simulink library "ESPA_lib"  (Simulink 7.5)
settings: Solver=ode45  StartTime=0.0  StopTime=10.0  RelTol=1e-3
values from neighbouring files (symbols this model uses):
  pESPA_bool_ToESPTrqSel_C = Simulink.Parameter    [ESPA_par.m]
  pESPA_cnt_TQDTrqDelyTi_C = Simulink.Parameter    [ESPA_par.m]
  pESPA_Nm_TMMinusTrq_C = Simulink.Parameter    [ESPA_par.m]
  pESPA_Nm_TMZeorTrq_C = Simulink.Parameter    [ESPA_par.m]
  pESPA_ratio_VehI_C = Simulink.Parameter    [ESPA_par.m]
  pESPA_rpm_TMZeroSpd_C = Simulink.Parameter    [ESPA_par.m]
libraries: BaseOperationLib_Browser x84
settings Model: Creator=wuaibin  LastModifiedBy=wuaibin

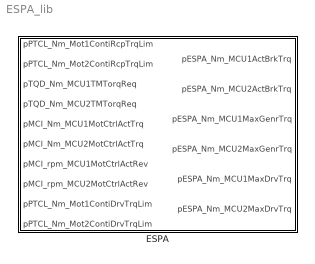
== system ESPA_lib ==
  ESPA : Subsystem

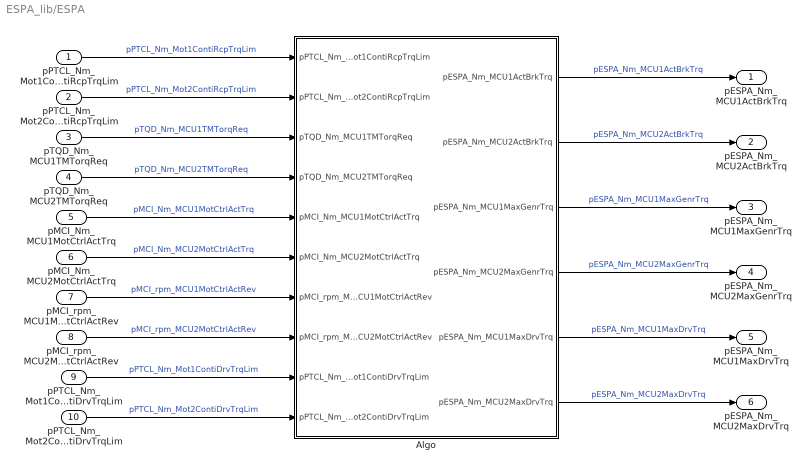
== system ESPA_lib/ESPA ==
  pPTCL_Nm_Mot1ContiRcpTrqLim : Inport
  pPTCL_Nm_Mot2ContiRcpTrqLim : Inport  Port=2
  pTQD_Nm_MCU1TMTorqReq : Inport  Port=3
  pTQD_Nm_MCU2TMTorqReq : Inport  Port=4
  pMCI_Nm_MCU1MotCtrlActTrq : Inport  Port=5
  pMCI_Nm_MCU2MotCtrlActTrq : Inport  Port=6
  pMCI_rpm_MCU1MotCtrlActRev : Inport  Port=7  OutDataType=fixdt(1, 16)  OutScaling=2^0
  pMCI_rpm_MCU2MotCtrlActRev : Inport  Port=8  OutDataType=fixdt(1, 16)  OutScaling=2^0
  pPTCL_Nm_Mot1ContiDrvTrqLim : Inport  Port=9
  pPTCL_Nm_Mot2ContiDrvTrqLim : Inport  Port=10
  Algo : Subsystem
  pESPA_Nm_MCU1ActBrkTrq : Outport  OutDataType=fixdt(1, 16)  OutScaling=2^0
  pESPA_Nm_MCU2ActBrkTrq : Outport  Port=2  OutDataType=fixdt(1, 16)  OutScaling=2^0
  pESPA_Nm_MCU1MaxGenrTrq : Outport  Port=3  OutDataType=fixdt(1, 16)  OutScaling=2^0
  pESPA_Nm_MCU2MaxGenrTrq : Outport  Port=4  OutDataType=fixdt(1, 16)  OutScaling=2^0
  pESPA_Nm_MCU1MaxDrvTrq : Outport  Port=5  OutDataType=fixdt(1, 16)  OutScaling=2^0
  pESPA_Nm_MCU2MaxDrvTrq : Outport  Port=6  OutDataType=fixdt(1, 16)  OutScaling=2^0
  wires:
  Algo/6(pESPA_Nm_MCU2MaxDrvTrq) -> pESPA_Nm_MCU2MaxDrvTrq/1  "pESPA_Nm_MCU2MaxDrvTrq"
  Algo/5(pESPA_Nm_MCU1MaxDrvTrq) -> pESPA_Nm_MCU1MaxDrvTrq/1  "pESPA_Nm_MCU1MaxDrvTrq"
  pPTCL_Nm_Mot2ContiDrvTrqLim/1 -> Algo/10(pPTCL_Nm_Mot2ContiDrvTrqLim)  "pPTCL_Nm_Mot2ContiDrvTrqLim"
  pPTCL_Nm_Mot1ContiDrvTrqLim/1 -> Algo/9(pPTCL_Nm_Mot1ContiDrvTrqLim)  "pPTCL_Nm_Mot1ContiDrvTrqLim"
  Algo/4(pESPA_Nm_MCU2MaxGenrTrq) -> pESPA_Nm_MCU2MaxGenrTrq/1  "pESPA_Nm_MCU2MaxGenrTrq"
  Algo/3(pESPA_Nm_MCU1MaxGenrTrq) -> pESPA_Nm_MCU1MaxGenrTrq/1  "pESPA_Nm_MCU1MaxGenrTrq"
  Algo/2(pESPA_Nm_MCU2ActBrkTrq) -> pESPA_Nm_MCU2ActBrkTrq/1  "pESPA_Nm_MCU2ActBrkTrq"
  Algo/1(pESPA_Nm_MCU1ActBrkTrq) -> pESPA_Nm_MCU1ActBrkTrq/1  "pESPA_Nm_MCU1ActBrkTrq"
  pTQD_Nm_MCU2TMTorqReq/1 -> Algo/4(pTQD_Nm_MCU2TMTorqReq)  "pTQD_Nm_MCU2TMTorqReq"
  pTQD_Nm_MCU1TMTorqReq/1 -> Algo/3(pTQD_Nm_MCU1TMTorqReq)  "pTQD_Nm_MCU1TMTorqReq"
  pPTCL_Nm_Mot2ContiRcpTrqLim/1 -> Algo/2(pPTCL_Nm_Mot2ContiRcpTrqLim)  "pPTCL_Nm_Mot2ContiRcpTrqLim"
  pPTCL_Nm_Mot1ContiRcpTrqLim/1 -> Algo/1(pPTCL_Nm_Mot1ContiRcpTrqLim)  "pPTCL_Nm_Mot1ContiRcpTrqLim"
  pMCI_rpm_MCU2MotCtrlActRev/1 -> Algo/8(pMCI_rpm_MCU2MotCtrlActRev)  "pMCI_rpm_MCU2MotCtrlActRev"
  pMCI_Nm_MCU1MotCtrlActTrq/1 -> Algo/5(pMCI_Nm_MCU1MotCtrlActTrq)  "pMCI_Nm_MCU1MotCtrlActTrq"
  pMCI_rpm_MCU1MotCtrlActRev/1 -> Algo/7(pMCI_rpm_MCU1MotCtrlActRev)  "pMCI_rpm_MCU1MotCtrlActRev"
  pMCI_Nm_MCU2MotCtrlActTrq/1 -> Algo/6(pMCI_Nm_MCU2MotCtrlActTrq)  "pMCI_Nm_MCU2MotCtrlActTrq"

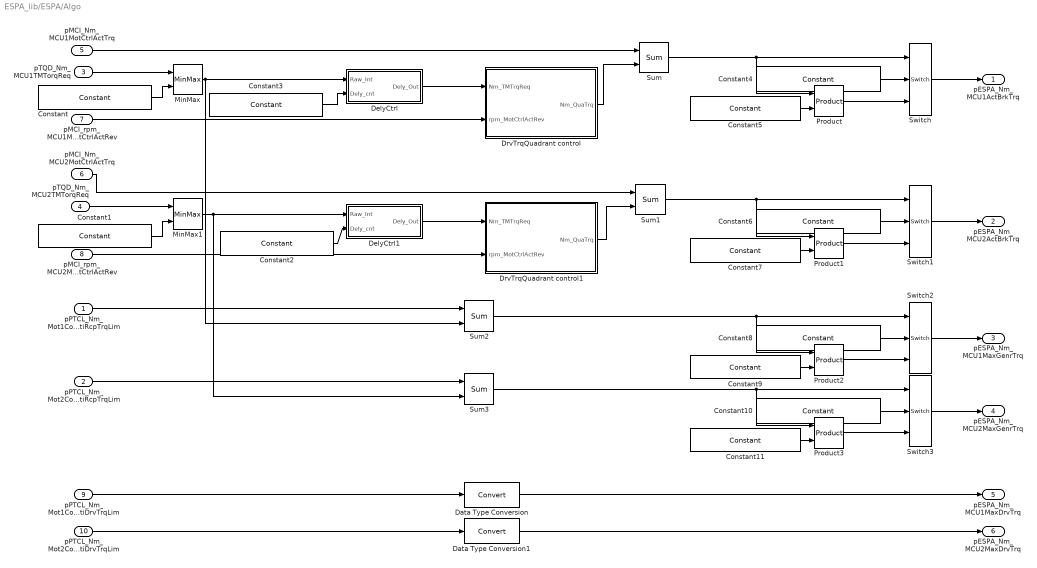
== system ESPA_lib/ESPA/Algo ==
  pPTCL_Nm_Mot1ContiRcpTrqLim : Inport
  pPTCL_Nm_Mot2ContiRcpTrqLim : Inport  Port=2
  pTQD_Nm_MCU1TMTorqReq : Inport  Port=3
  pTQD_Nm_MCU2TMTorqReq : Inport  Port=4
  pMCI_Nm_MCU1MotCtrlActTrq : Inport  Port=5
  pMCI_Nm_MCU2MotCtrlActTrq : Inport  Port=6
  pMCI_rpm_MCU1MotCtrlActRev : Inport  Port=7  OutDataType=fixdt(1, 16)  OutScaling=2^0
  pMCI_rpm_MCU2MotCtrlActRev : Inport  Port=8  OutDataType=fixdt(1, 16)  OutScaling=2^0
  pPTCL_Nm_Mot1ContiDrvTrqLim : Inport  Port=9
  pPTCL_Nm_Mot2ContiDrvTrqLim : Inport  Port=10
  Constant : BaseOperationLib_Browser/Sources&Sinks/Constant  Value=pESPA_Nm_TMZeorTrq_C  OutMin=[]  OutMax=[]  OutDataType=fixdt(1, 16)  ConRadixGroup=Use specified scaling  OutScaling=2^0  OutDataTypeStr=Inherit: Inherit from 'Constant value'
  Constant1 : BaseOperationLib_Browser/Sources&Sinks/Constant  Value=pESPA_Nm_TMZeorTrq_C  OutMin=[]  OutMax=[]  OutDataType=fixdt(1, 16)  ConRadixGroup=Use specified scaling  OutScaling=2^0  OutDataTypeStr=Inherit: Inherit from 'Constant value'
  Constant{4,6,8,10} (4 alike) : BaseOperationLib_Browser/Sources&Sinks/Constant  Value=pESPA_bool_ToESPTrqSel_C  OutMin=[]  OutMax=[]  OutDataType=fixdt(1, 16)  ConRadixGroup=Use specified scaling  OutScaling=2^0  OutDataTypeStr=Inherit: Inherit from 'Constant value'
  Constant{5,7,9,11} (4 alike) : BaseOperationLib_Browser/Sources&Sinks/Constant  Value=pESPA_ratio_VehI_C  OutMin=[]  OutMax=[]  OutDataType=fixdt(1, 16)  ConRadixGroup=Use specified scaling  OutScaling=2^0  OutDataTypeStr=Inherit: Inherit from 'Constant value'
  Constant2 : BaseOperationLib_Browser/Sources&Sinks/Constant  Value=pESPA_cnt_TQDTrqDelyTi_C  OutMin=[]  OutMax=[]  OutDataType=fixdt(1, 16)  ConRadixGroup=Use specified scaling  OutScaling=2^0  OutDataTypeStr=Inherit: Inherit from 'Constant value'
  Constant3 : BaseOperationLib_Browser/Sources&Sinks/Constant  Value=pESPA_cnt_TQDTrqDelyTi_C  OutMin=[]  OutMax=[]  OutDataType=fixdt(1, 16)  ConRadixGroup=Use specified scaling  OutScaling=2^0  OutDataTypeStr=Inherit: Inherit from 'Constant value'
  Data Type Conversion : DataTypeConversion  OutDataType=fixdt(1, 16)  OutScaling=2^0
  Data Type Conversion1 : DataTypeConversion  OutDataType=fixdt(1, 16)  OutScaling=2^0
  DelyCtrl : Subsystem
  DelyCtrl1 : Subsystem
  DrvTrqQuadrant control : Subsystem
  DrvTrqQuadrant control1 : Subsystem
  MinMax : BaseOperationLib_Browser/Math Operations Changed/MinMax  Function=min  Inputs=2  InputSameDT=on  OutMin=[]  OutMax=[]  OutDataType=fixdt(1, 16)  OutScaling=2^0  SaturateOnIntegerOverflow=on
  MinMax1 : BaseOperationLib_Browser/Math Operations Changed/MinMax  Function=min  Inputs=2  InputSameDT=on  OutMin=[]  OutMax=[]  OutDataType=fixdt(1, 16)  OutScaling=2^0  SaturateOnIntegerOverflow=on
  Product{,1..3} (4 alike) : BaseOperationLib_Browser/Math Operations Changed/Product  Inputs=2  Multiplication=Element-wise(.*)  OutMin=[]  OutMax=[]  OutDataType=fixdt(1,16,0)  OutScaling=[]  OutDataTypeStr=Inherit: Inherit via back propagation  RndMeth=Zero  SaturateOnIntegerOverflow=on
  Sum{,1..3} (4 alike) : BaseOperationLib_Browser/Math Operations Changed/Sum  Inputs=+-  InputSameDT=on  OutMin=[]  OutMax=[]  OutDataType=fixdt(1, 16)  OutScaling=2^0  SaturateOnIntegerOverflow=on
  Switch{,1..3} (4 alike) : BaseOperationLib_Browser/Signal Routing Changed/Switch  Criteria=u2 ~= 0  Threshold=1  InputSameDT=on  OutMin=[]  OutMax=[]  OutDataType=fixdt(1,16,0)  OutScaling=[]  SaturateOnIntegerOverflow=on
  pESPA_Nm_MCU1ActBrkTrq : Outport  OutDataType=fixdt(1, 16)  OutScaling=2^0
  pESPA_Nm_MCU2ActBrkTrq : Outport  Port=2  OutDataType=fixdt(1, 16)  OutScaling=2^0
  pESPA_Nm_MCU1MaxGenrTrq : Outport  Port=3  OutDataType=fixdt(1, 16)  OutScaling=2^0
  pESPA_Nm_MCU2MaxGenrTrq : Outport  Port=4  OutDataType=fixdt(1, 16)  OutScaling=2^0
  pESPA_Nm_MCU1MaxDrvTrq : Outport  Port=5  OutDataType=fixdt(1, 16)  OutScaling=2^0
  pESPA_Nm_MCU2MaxDrvTrq : Outport  Port=6  OutDataType=fixdt(1, 16)  OutScaling=2^0
  wires:
  Constant3/1 -> DelyCtrl/2(Dely_cnt)
  Constant2/1 -> DelyCtrl1/2(Dely_cnt)
  pPTCL_Nm_Mot2ContiDrvTrqLim/1 -> Data Type Conversion1/1
  pPTCL_Nm_Mot1ContiDrvTrqLim/1 -> Data Type Conversion/1
  pPTCL_Nm_Mot2ContiRcpTrqLim/1 -> Sum3/1
  pPTCL_Nm_Mot1ContiRcpTrqLim/1 -> Sum2/1
  Constant1/1 -> MinMax1/2
  Constant/1 -> MinMax/2
  DrvTrqQuadrant control1/1(Nm_QuaTrq) -> Sum1/2
  pMCI_Nm_MCU1MotCtrlActTrq/1 -> Sum/1
  DrvTrqQuadrant control/1(Nm_QuaTrq) -> Sum/2
  pMCI_rpm_MCU2MotCtrlActRev/1 -> DrvTrqQuadrant control1/2(rpm_MotCtrlActRev)
  pMCI_rpm_MCU1MotCtrlActRev/1 -> DrvTrqQuadrant control/2(rpm_MotCtrlActRev)
  pMCI_Nm_MCU2MotCtrlActTrq/1 -> Sum1/1
  pTQD_Nm_MCU1TMTorqReq/1 -> MinMax/1
  MinMax/1 -> DelyCtrl/1(Raw_Int), Sum2/2
  DelyCtrl/1(Dely_Out) -> DrvTrqQuadrant control/1(Nm_TMTrqReq)
  pTQD_Nm_MCU2TMTorqReq/1 -> MinMax1/1
  MinMax1/1 -> DelyCtrl1/1(Raw_Int), Sum3/2
  DelyCtrl1/1(Dely_Out) -> DrvTrqQuadrant control1/1(Nm_TMTrqReq)
  Data Type Conversion1/1 -> pESPA_Nm_MCU2MaxDrvTrq/1
  Data Type Conversion/1 -> pESPA_Nm_MCU1MaxDrvTrq/1
  Constant4/1 -> Switch/2
  Sum/1 -> Switch/1, Product/1
  Switch/1 -> pESPA_Nm_MCU1ActBrkTrq/1
  Product/1 -> Switch/3
  Constant5/1 -> Product/2
  Constant6/1 -> Switch1/2
  Sum1/1 -> Product1/1, Switch1/1
  Product1/1 -> Switch1/3
  Constant7/1 -> Product1/2
  Switch1/1 -> pESPA_Nm_MCU2ActBrkTrq/1
  Constant8/1 -> Switch2/2
  Sum2/1 -> Switch2/1, Product2/1
  Product2/1 -> Switch2/3
  Constant9/1 -> Product2/2
  Switch2/1 -> pESPA_Nm_MCU1MaxGenrTrq/1
  Constant10/1 -> Switch3/2
  Sum3/1 -> Product3/1, Switch3/1
  Product3/1 -> Switch3/3
  Constant11/1 -> Product3/2
  Switch3/1 -> pESPA_Nm_MCU2MaxGenrTrq/1

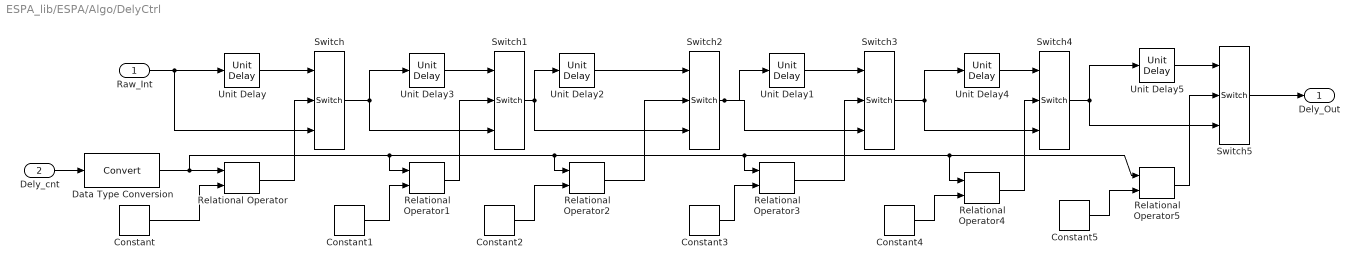
== system ESPA_lib/ESPA/Algo/DelyCtrl ==
  Raw_Int : Inport  OutDataType=fixdt(1, 16)  OutScaling=2^0
  Dely_cnt : Inport  Port=2  OutDataType=fixdt(1, 16)  OutScaling=2^0
  Constant : BaseOperationLib_Browser/Sources&Sinks/Constant  Value=1  OutMin=[]  OutMax=[]  OutDataType=fixdt(1, 16)  ConRadixGroup=Use specified scaling  OutScaling=2^0  OutDataTypeStr=Inherit: Inherit from 'Constant value'
  Constant1 : BaseOperationLib_Browser/Sources&Sinks/Constant  Value=2  OutMin=[]  OutMax=[]  OutDataType=fixdt(1, 16)  ConRadixGroup=Use specified scaling  OutScaling=2^0  OutDataTypeStr=Inherit: Inherit from 'Constant value'
  Constant2 : BaseOperationLib_Browser/Sources&Sinks/Constant  Value=3  OutMin=[]  OutMax=[]  OutDataType=fixdt(1, 16)  ConRadixGroup=Use specified scaling  OutScaling=2^0  OutDataTypeStr=Inherit: Inherit from 'Constant value'
  Constant3 : BaseOperationLib_Browser/Sources&Sinks/Constant  Value=4  OutMin=[]  OutMax=[]  OutDataType=fixdt(1, 16)  ConRadixGroup=Use specified scaling  OutScaling=2^0  OutDataTypeStr=Inherit: Inherit from 'Constant value'
  Constant4 : BaseOperationLib_Browser/Sources&Sinks/Constant  Value=5  OutMin=[]  OutMax=[]  OutDataType=fixdt(1, 16)  ConRadixGroup=Use specified scaling  OutScaling=2^0  OutDataTypeStr=Inherit: Inherit from 'Constant value'
  Constant5 : BaseOperationLib_Browser/Sources&Sinks/Constant  Value=6  OutMin=[]  OutMax=[]  OutDataType=fixdt(1, 16)  ConRadixGroup=Use specified scaling  OutScaling=2^0  OutDataTypeStr=Inherit: Inherit from 'Constant value'
  Data Type Conversion : DataTypeConversion  OutDataType=fixdt(1, 16)  OutScaling=2^0
  Relational Operator{,1..5} (6 alike) : BaseOperationLib_Browser/Logic Operations Changed/Relational Operator  Operator=>=  InputSameDT=on  LogicOutDataTypeMode=Specify via dialog  LogicDataType=PDT_Bool  OutDataTypeStr=PDT_Bool
  Switch{,1..5} (6 alike) : BaseOperationLib_Browser/Signal Routing Changed/Switch  Criteria=u2 ~= 0  Threshold=1  InputSameDT=on  OutMin=[]  OutMax=[]  OutDataType=fixdt(1,16,0)  OutScaling=[]  SaturateOnIntegerOverflow=on
  Unit Delay{,1..5} (6 alike) : BaseOperationLib_Browser/Discrete Unchanged /Unit Delay  X0=0  SampleTime=-1
  Dely_Out : Outport  OutDataType=fixdt(1, 16)  OutScaling=2^0
  wires:
  Data Type Conversion/1 -> Relational Operator2/1, Relational Operator3/1, Relational Operator4/1, Relational Operator5/1, Relational Operator1/1, Relational Operator/1
  Constant3/1 -> Relational Operator3/2
  Unit Delay1/1 -> Switch3/1
  Switch2/1 -> Unit Delay1/1, Switch3/3
  Relational Operator2/1 -> Switch2/2
  Constant2/1 -> Relational Operator2/2
  Relational Operator1/1 -> Switch1/2
  Constant1/1 -> Relational Operator1/2
  Constant/1 -> Relational Operator/2
  Dely_cnt/1 -> Data Type Conversion/1
  Relational Operator/1 -> Switch/2
  Unit Delay2/1 -> Switch2/1
  Switch1/1 -> Switch2/3, Unit Delay2/1
  Unit Delay3/1 -> Switch1/1
  Switch/1 -> Switch1/3, Unit Delay3/1
  Raw_Int/1 -> Switch/3, Unit Delay/1
  Unit Delay/1 -> Switch/1
  Switch3/1 -> Unit Delay4/1, Switch4/3
  Unit Delay4/1 -> Switch4/1
  Constant4/1 -> Relational Operator4/2
  Relational Operator4/1 -> Switch4/2
  Switch4/1 -> Switch5/3, Unit Delay5/1
  Unit Delay5/1 -> Switch5/1
  Constant5/1 -> Relational Operator5/2
  Relational Operator5/1 -> Switch5/2
  Relational Operator3/1 -> Switch3/2
  Switch5/1 -> Dely_Out/1

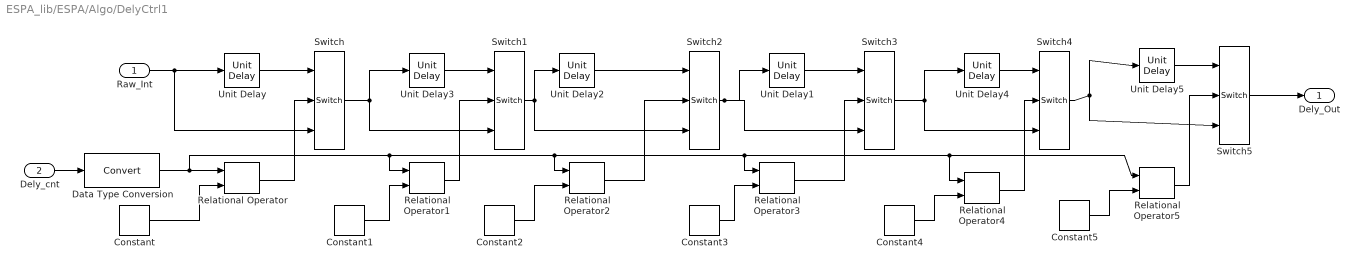
== system ESPA_lib/ESPA/Algo/DelyCtrl1 ==
  Raw_Int : Inport  OutDataType=fixdt(1, 16)  OutScaling=2^0
  Dely_cnt : Inport  Port=2  OutDataType=fixdt(1, 16)  OutScaling=2^0
  Constant : BaseOperationLib_Browser/Sources&Sinks/Constant  Value=1  OutMin=[]  OutMax=[]  OutDataType=fixdt(1, 16)  ConRadixGroup=Use specified scaling  OutScaling=2^0  OutDataTypeStr=Inherit: Inherit from 'Constant value'
  Constant1 : BaseOperationLib_Browser/Sources&Sinks/Constant  Value=2  OutMin=[]  OutMax=[]  OutDataType=fixdt(1, 16)  ConRadixGroup=Use specified scaling  OutScaling=2^0  OutDataTypeStr=Inherit: Inherit from 'Constant value'
  Constant2 : BaseOperationLib_Browser/Sources&Sinks/Constant  Value=3  OutMin=[]  OutMax=[]  OutDataType=fixdt(1, 16)  ConRadixGroup=Use specified scaling  OutScaling=2^0  OutDataTypeStr=Inherit: Inherit from 'Constant value'
  Constant3 : BaseOperationLib_Browser/Sources&Sinks/Constant  Value=4  OutMin=[]  OutMax=[]  OutDataType=fixdt(1, 16)  ConRadixGroup=Use specified scaling  OutScaling=2^0  OutDataTypeStr=Inherit: Inherit from 'Constant value'
  Constant4 : BaseOperationLib_Browser/Sources&Sinks/Constant  Value=5  OutMin=[]  OutMax=[]  OutDataType=fixdt(1, 16)  ConRadixGroup=Use specified scaling  OutScaling=2^0  OutDataTypeStr=Inherit: Inherit from 'Constant value'
  Constant5 : BaseOperationLib_Browser/Sources&Sinks/Constant  Value=6  OutMin=[]  OutMax=[]  OutDataType=fixdt(1, 16)  ConRadixGroup=Use specified scaling  OutScaling=2^0  OutDataTypeStr=Inherit: Inherit from 'Constant value'
  Data Type Conversion : DataTypeConversion  OutDataType=fixdt(1, 16)  OutScaling=2^0
  Relational Operator{,1..5} (6 alike) : BaseOperationLib_Browser/Logic Operations Changed/Relational Operator  Operator=>=  InputSameDT=on  LogicOutDataTypeMode=Specify via dialog  LogicDataType=PDT_Bool  OutDataTypeStr=PDT_Bool
  Switch{,1..5} (6 alike) : BaseOperationLib_Browser/Signal Routing Changed/Switch  Criteria=u2 ~= 0  Threshold=1  InputSameDT=on  OutMin=[]  OutMax=[]  OutDataType=fixdt(1,16,0)  OutScaling=[]  SaturateOnIntegerOverflow=on
  Unit Delay{,1..5} (6 alike) : BaseOperationLib_Browser/Discrete Unchanged /Unit Delay  X0=0  SampleTime=-1
  Dely_Out : Outport  OutDataType=fixdt(1, 16)  OutScaling=2^0
  wires:
  Switch5/1 -> Dely_Out/1
  Relational Operator3/1 -> Switch3/2
  Relational Operator5/1 -> Switch5/2
  Constant5/1 -> Relational Operator5/2
  Unit Delay5/1 -> Switch5/1
  Switch4/1 -> Unit Delay5/1, Switch5/3
  Relational Operator4/1 -> Switch4/2
  Constant4/1 -> Relational Operator4/2
  Unit Delay4/1 -> Switch4/1
  Switch3/1 -> Switch4/3, Unit Delay4/1
  Unit Delay/1 -> Switch/1
  Raw_Int/1 -> Unit Delay/1, Switch/3
  Switch/1 -> Unit Delay3/1, Switch1/3
  Unit Delay3/1 -> Switch1/1
  Switch1/1 -> Unit Delay2/1, Switch2/3
  Unit Delay2/1 -> Switch2/1
  Relational Operator/1 -> Switch/2
  Dely_cnt/1 -> Data Type Conversion/1
  Constant/1 -> Relational Operator/2
  Constant1/1 -> Relational Operator1/2
  Relational Operator1/1 -> Switch1/2
  Constant2/1 -> Relational Operator2/2
  Relational Operator2/1 -> Switch2/2
  Switch2/1 -> Switch3/3, Unit Delay1/1
  Unit Delay1/1 -> Switch3/1
  Constant3/1 -> Relational Operator3/2
  Data Type Conversion/1 -> Relational Operator/1, Relational Operator1/1, Relational Operator5/1, Relational Operator4/1, Relational Operator3/1, Relational Operator2/1

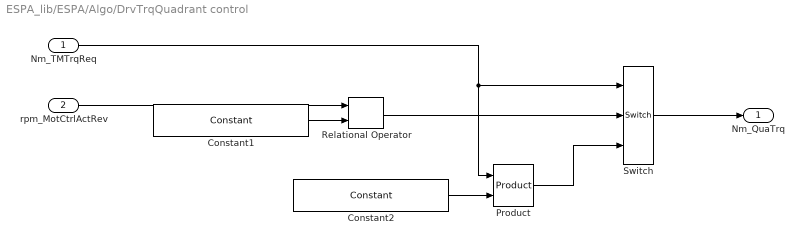
== system ESPA_lib/ESPA/Algo/DrvTrqQuadrant control ==
  Nm_TMTrqReq : Inport
  rpm_MotCtrlActRev : Inport  Port=2
  Constant1 : BaseOperationLib_Browser/Sources&Sinks/Constant  Value=pESPA_rpm_TMZeroSpd_C  OutMin=[]  OutMax=[]  OutDataType=fixdt(1, 16)  ConRadixGroup=Use specified scaling  OutScaling=2^0  OutDataTypeStr=Inherit: Inherit from 'Constant value'
  Constant2 : BaseOperationLib_Browser/Sources&Sinks/Constant  Value=pESPA_Nm_TMMinusTrq_C  OutMin=[]  OutMax=[]  OutDataType=fixdt(1, 16)  ConRadixGroup=Use specified scaling  OutScaling=2^0  OutDataTypeStr=Inherit: Inherit from 'Constant value'
  Product : BaseOperationLib_Browser/Math Operations Changed/Product  Inputs=2  Multiplication=Element-wise(.*)  OutMin=[]  OutMax=[]  OutDataType=fixdt(1,16,0)  OutScaling=[]  OutDataTypeStr=Inherit: Inherit via back propagation  RndMeth=Zero  SaturateOnIntegerOverflow=on
  Relational Operator : BaseOperationLib_Browser/Logic Operations Changed/Relational Operator  Operator=>=  InputSameDT=on  LogicOutDataTypeMode=Specify via dialog  LogicDataType=PDT_Bool  OutDataTypeStr=PDT_Bool
  Switch : BaseOperationLib_Browser/Signal Routing Changed/Switch  Criteria=u2 ~= 0  Threshold=1  InputSameDT=on  OutMin=[]  OutMax=[]  OutDataType=fixdt(1,16,0)  OutScaling=[]  SaturateOnIntegerOverflow=on
  Nm_QuaTrq : Outport
  wires:
  Switch/1 -> Nm_QuaTrq/1
  rpm_MotCtrlActRev/1 -> Relational Operator/1
  Nm_TMTrqReq/1 -> Switch/1, Product/1
  Product/1 -> Switch/3
  Constant2/1 -> Product/2
  Relational Operator/1 -> Switch/2
  Constant1/1 -> Relational Operator/2

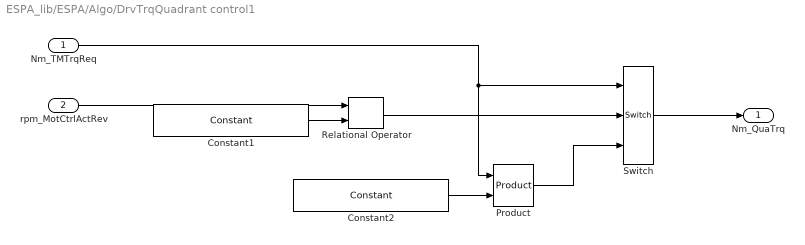
== system ESPA_lib/ESPA/Algo/DrvTrqQuadrant control1 ==
  Nm_TMTrqReq : Inport
  rpm_MotCtrlActRev : Inport  Port=2
  Constant1 : BaseOperationLib_Browser/Sources&Sinks/Constant  Value=pESPA_rpm_TMZeroSpd_C  OutMin=[]  OutMax=[]  OutDataType=fixdt(1, 16)  ConRadixGroup=Use specified scaling  OutScaling=2^0  OutDataTypeStr=Inherit: Inherit from 'Constant value'
  Constant2 : BaseOperationLib_Browser/Sources&Sinks/Constant  Value=pESPA_Nm_TMMinusTrq_C  OutMin=[]  OutMax=[]  OutDataType=fixdt(1, 16)  ConRadixGroup=Use specified scaling  OutScaling=2^0  OutDataTypeStr=Inherit: Inherit from 'Constant value'
  Product : BaseOperationLib_Browser/Math Operations Changed/Product  Inputs=2  Multiplication=Element-wise(.*)  OutMin=[]  OutMax=[]  OutDataType=fixdt(1,16,0)  OutScaling=[]  OutDataTypeStr=Inherit: Inherit via back propagation  RndMeth=Zero  SaturateOnIntegerOverflow=on
  Relational Operator : BaseOperationLib_Browser/Logic Operations Changed/Relational Operator  Operator=>=  InputSameDT=on  LogicOutDataTypeMode=Specify via dialog  LogicDataType=PDT_Bool  OutDataTypeStr=PDT_Bool
  Switch : BaseOperationLib_Browser/Signal Routing Changed/Switch  Criteria=u2 ~= 0  Threshold=1  InputSameDT=on  OutMin=[]  OutMax=[]  OutDataType=fixdt(1,16,0)  OutScaling=[]  SaturateOnIntegerOverflow=on
  Nm_QuaTrq : Outport
  wires:
  Constant1/1 -> Relational Operator/2
  Relational Operator/1 -> Switch/2
  Constant2/1 -> Product/2
  Product/1 -> Switch/3
  Nm_TMTrqReq/1 -> Product/1, Switch/1
  rpm_MotCtrlActRev/1 -> Relational Operator/1
  Switch/1 -> Nm_QuaTrq/1
